simulink model "QuadCopter"  (R2016a)
settings: Solver=ode23t  StartTime=0.0  StopTime=12  FixedStep=0.001  RelTol=1e-5
InitFcn:
  | %load QuadCopterParameters
values from neighbouring files (symbols this model uses):
  Mass = 0.458    [QuadCopterParameters_m.m]
  motorCoeffs = [0.00010909388854752541 0.0075590948720063037 0.09060950915942291                 ]    [QuadCopterParameters_m.m]
undefined symbols (not defined in the file or in its folder): dc, g, Motor_F, Mxfactor, Myfactor, Qlx, Qly
libraries: Lib_Sensors x3, aerolibobsolete x1, simulink x1
settings Model: Creator=rruff  LastModifiedBy=Administrator
settings DataIOCC: LimitDataPoints=on  SaveFormat=Array  SaveOutput=off  SaveTime=off
settings OptimizationCC: DefaultParameterBehavior=Inlined  ExpressionDepthLimit=2147483647
settings DebuggingCC: SignalInfNanChecking=error  AlgebraicLoopMsg=error  UnderspecifiedInitializationDetection=Classic  MergeDetectMultiDrivingBlocksExec=none  MultiTaskDSMMsg=warning  MultiTaskCondExecSysMsg=none  FcnCallInpInsideContextMsg=EnableAllAsWarning  UnconnectedInputMsg=none  UnconnectedOutputMsg=none  UnconnectedLineMsg=none  StateNameClashWarn=warning
settings HardwareCC: ProdBitPerPointer=32  ProdLargestAtomicFloat=None  ProdIntDivRoundTo=Undefined  ProdEndianess=Unspecified  ProdWordSize=32  ProdHWDeviceType=Generic->32-bit Embedded Processor
settings ModelReferenceCC: ModelReferenceNumInstancesAllowed=Single  PropagateSignalLabelsOutOfModel=off
settings ConfigComp: CovModelRefEnable=Off  CovSFcnEnable=off
settings SimscapeCC: SelectedTab=SimMechanics2G
settings SimMechanicsCC: VisOnUpdateDiagram=on  VisDuringSimulation=on  FramesToBeSkipped=10  AnimationDelay=0  LastVizWinPosition=[1022 659 560 420]  CamPosition=[10.2752;-3.21889;-2.95529;]  CamTarget=[0;-2.23517e-09;-0.0242675;]  CamUpVector=[-0.23308;0.133123;-0.963303;]  CamHeight=0.224542  VisBackgroundColor=[0.9;0.9;0.95;]  DefaultBodyColor=[1;0;0;]
settings ConfigurationSet: Description=SimMechanics 2G
settings ExplorerConfigSet: SimMechanicsOpenEditorOnUpdate=off

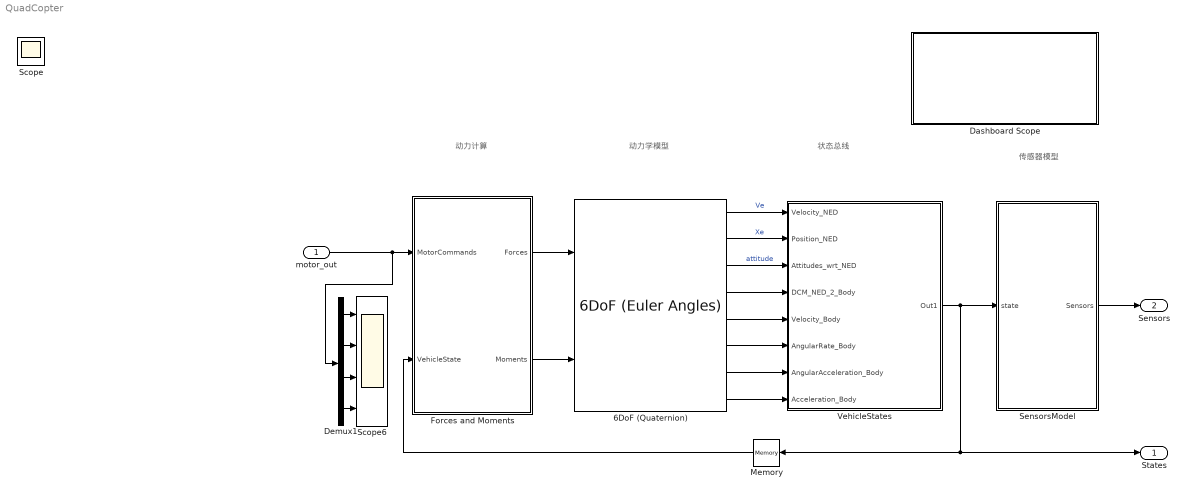
== system QuadCopter ==
  note: 传感器模型
  note: 状态总线
  note: 动力学模型
  note: 动力计算
  motor_out : Inport  PortDimensions=[4,1]
  6DoF (Quaternion) : aerolibobsolete/6DoF (Euler Angles)  units=Metric (MKS)  mtype=Fixed  rep=Quaternion  xme_0=[0 0 0]  Vm_0=[0 0 0]  eul_0=[0 0 0]  pm_0=[0 0 0]  mass_0=Mass  mass_e=0  mass_f=0  inertia=MomentInertiaTensor  inertia_e=eye(3)  inertia_f=eye(3)  k_quat=1.0
  Dashboard Scope : Subsystem  DialogController=hmiCreateDDGDialog  IsWebBlock=on  mask(MWDashboardBlock){webBlockId=dbd7d4e6-1bb4-4b4b-bc68-27a6a6e553e4, webBlockType=sdiscope, ShowInitialText=on, HMISrcModelName=QuadCopter}
      mask prompts: webBlockId "WebBlock Id"; webBlockType "WebBlock Type"; HMISrcModelName "Source Model"
      mask Help: helpview([docroot '/mapfiles/simulink.map'], 'hmi_scope')
      mask Display:
      | if strcmp(get_param(bdroot(gcb),'BlockDiagramType'), 'library')
      |     image([(matlabroot) '/toolbox/simulink/hmi/icons/DashboardScope.png']);
      | end
  Demux1 : Demux
  Forces and Moments : Subsystem  TreatAsAtomicUnit=on
  Memory : Memory
  Scope6 : Scope  NumInputPorts=4
  SensorsModel : Subsystem
  VehicleStates : Subsystem
  States : Outport  OutDataTypeStr=Bus: VehicleStates
  Sensors : Outport  Port=2  OutDataTypeStr=Bus: Sensors
  Scope : Scope
  wires:
  6DoF (Quaternion)/6 -> VehicleStates/6(AngularRate_Body)
  6DoF (Quaternion)/8 -> VehicleStates/8(Acceleration_Body)
  6DoF (Quaternion)/4 -> VehicleStates/4(DCM_NED_2_Body)
  6DoF (Quaternion)/5 -> VehicleStates/5(Velocity_Body)
  6DoF (Quaternion)/7 -> VehicleStates/7(AngularAcceleration_Body)
  6DoF (Quaternion)/3 -> VehicleStates/3(Attitudes_wrt_NED)  "attitude"
  6DoF (Quaternion)/1 -> VehicleStates/1(Velocity_NED)  "Ve"
  VehicleStates/1(Out1) -> SensorsModel/1(state), States/1, Memory/1
  6DoF (Quaternion)/2 -> VehicleStates/2(Position_NED)  "Xe"
  Memory/1 -> Forces and Moments/2(VehicleState)
  Forces and Moments/1(Forces) -> 6DoF (Quaternion)/1
  Forces and Moments/2(Moments) -> 6DoF (Quaternion)/2
  Demux1/1 -> Scope6/1
  Demux1/2 -> Scope6/2
  Demux1/3 -> Scope6/3
  Demux1/4 -> Scope6/4
  motor_out/1 -> Demux1/1, Forces and Moments/1(MotorCommands)
  SensorsModel/1(Sensors) -> Sensors/1

== system QuadCopter/Dashboard Scope ==

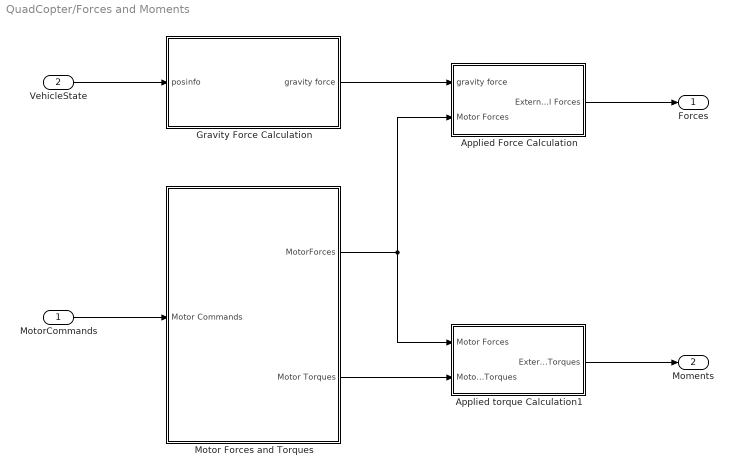
== system QuadCopter/Forces and Moments ==
  MotorCommands : Inport
  VehicleState : Inport  Port=2
  Applied Force Calculation : Subsystem
  Applied torque Calculation1 : Subsystem
  Gravity Force Calculation : Subsystem
  Motor Forces and Torques : Subsystem
  Forces : Outport
  Moments : Outport  Port=2
  wires:
  Motor Forces and Torques/1(MotorForces) -> Applied torque Calculation1/1(Motor Forces), Applied Force Calculation/2(Motor Forces)
  Applied Force Calculation/1(External Forces) -> Forces/1
  Motor Forces and Torques/2(Motor Torques) -> Applied torque Calculation1/2(Motor Torques)
  Applied torque Calculation1/1(External Torques) -> Moments/1
  MotorCommands/1 -> Motor Forces and Torques/1(Motor Commands)
  VehicleState/1 -> Gravity Force Calculation/1(posinfo)
  Gravity Force Calculation/1(gravity force) -> Applied Force Calculation/1(gravity force)

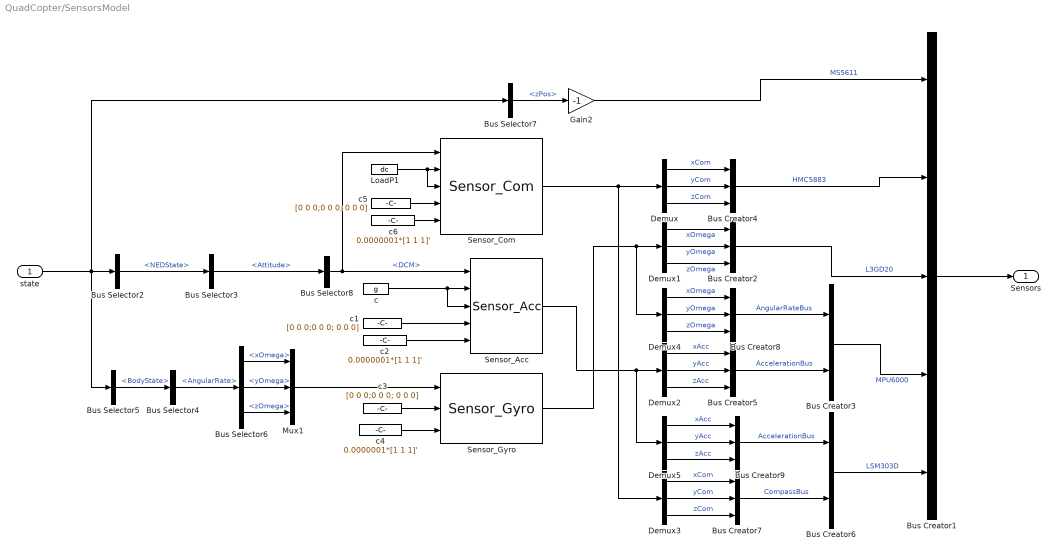
== system QuadCopter/SensorsModel ==
  state : Inport
  Bus Creator1 : BusCreator  Inputs=5  OutDataTypeStr=Bus: Sensors  NonVirtualBus=on
  Bus Creator2 : BusCreator  Inputs=3  OutDataTypeStr=Bus: AngularRateBus  NonVirtualBus=on
  Bus Creator3 : BusCreator  Inputs=2  OutDataTypeStr=Bus: MPU6000  NonVirtualBus=on
  Bus Creator4 : BusCreator  Inputs=3  OutDataTypeStr=Bus: CompassBus  NonVirtualBus=on
  Bus Creator5 : BusCreator  Inputs=3  OutDataTypeStr=Bus: AccelerationBus  NonVirtualBus=on
  Bus Creator6 : BusCreator  Inputs=2  OutDataTypeStr=Bus: LSM303D  NonVirtualBus=on
  Bus Creator7 : BusCreator  Inputs=3  OutDataTypeStr=Bus: CompassBus  NonVirtualBus=on
  Bus Creator8 : BusCreator  Inputs=3  OutDataTypeStr=Bus: AngularRateBus  NonVirtualBus=on
  Bus Creator9 : BusCreator  Inputs=3  OutDataTypeStr=Bus: AccelerationBus  NonVirtualBus=on
  Bus Selector2 : BusSelector  OutputSignals=NEDState
  Bus Selector3 : BusSelector  OutputSignals=Attitude
  Bus Selector4 : BusSelector  OutputSignals=AngularRate
  Bus Selector5 : BusSelector  OutputSignals=BodyState
  Bus Selector6 : BusSelector  OutputSignals=xOmega,yOmega,zOmega
  Bus Selector7 : BusSelector  OutputSignals=NEDState.Position.zPos
  Bus Selector8 : BusSelector  OutputSignals=DCM
  Demux{,1..5} (6 alike) : Demux  Outputs=3
  Gain2 : Gain  Gain=-1
  LoadP1 : Constant  Value=dc  SampleTime=0
  Mux1 : Mux  Inputs=3
  Sensor_Acc : Lib_Sensors/Sensor_Acc
  Sensor_Com : Lib_Sensors/Sensor_Com
  Sensor_Gyro : Lib_Sensors/Sensor_Gyro
  c : Constant  Value=g  SampleTime=0
  c1 : Constant  Value=[0 0 0;0 0 0; 0 0 0]  SampleTime=0
  c2 : Constant  Value=0.0000001*[1 1 1]'  SampleTime=0
  c3 : Constant  Value=[0 0 0;0 0 0; 0 0 0]  SampleTime=0
  c4 : Constant  Value=0.0000001*[1 1 1]'  SampleTime=0
  c5 : Constant  Value=[0 0 0;0 0 0; 0 0 0]  SampleTime=0
  c6 : Constant  Value=0.0000001*[1 1 1]'  SampleTime=0
  Sensors : Outport  OutDataTypeStr=Bus: Sensors
  wires:
  state/1 -> Bus Selector2/1, Bus Selector7/1, Bus Selector5/1
  Bus Selector2/1 -> Bus Selector3/1  "<NEDState>"
  Bus Selector5/1 -> Bus Selector4/1  "<BodyState>"
  Bus Selector4/1 -> Bus Selector6/1  "<AngularRate>"
  LoadP1/1 -> Sensor_Com/3, Sensor_Com/2
  Bus Selector6/2 -> Mux1/2  "<yOmega>"
  Bus Selector6/3 -> Mux1/3  "<zOmega>"
  Bus Selector3/1 -> Bus Selector8/1  "<Attitude>"
  Bus Selector6/1 -> Mux1/1  "<xOmega>"
  Gain2/1 -> Bus Creator1/1  "MS5611"
  Bus Creator3/1 -> Bus Creator1/4  "MPU6000"
  Bus Creator6/1 -> Bus Creator1/5  "LSM303D"
  Demux/1 -> Bus Creator4/1  "xCom"
  Demux/2 -> Bus Creator4/2  "yCom"
  Demux/3 -> Bus Creator4/3  "zCom"
  Sensor_Com/1 -> Demux3/1, Demux/1
  Demux1/1 -> Bus Creator2/1  "xOmega"
  Demux1/2 -> Bus Creator2/2  "yOmega"
  Demux1/3 -> Bus Creator2/3  "zOmega"
  Sensor_Gyro/1 -> Demux1/1, Demux4/1
  Bus Creator5/1 -> Bus Creator3/2  "AccelerationBus"
  Demux2/1 -> Bus Creator5/1  "xAcc"
  Demux2/2 -> Bus Creator5/2  "yAcc"
  Demux2/3 -> Bus Creator5/3  "zAcc"
  Bus Creator2/1 -> Bus Creator1/3  "L3GD20"
  Bus Creator4/1 -> Bus Creator1/2  "HMC5883"
  Demux3/1 -> Bus Creator7/1  "xCom"
  Demux3/2 -> Bus Creator7/2  "yCom"
  Demux3/3 -> Bus Creator7/3  "zCom"
  Bus Creator7/1 -> Bus Creator6/2  "CompassBus"
  Bus Creator1/1 -> Sensors/1
  Demux4/1 -> Bus Creator8/1  "xOmega"
  Demux4/2 -> Bus Creator8/2  "yOmega"
  Demux4/3 -> Bus Creator8/3  "zOmega"
  Bus Creator8/1 -> Bus Creator3/1  "AngularRateBus"
  Demux5/1 -> Bus Creator9/1  "xAcc"
  Demux5/2 -> Bus Creator9/2  "yAcc"
  Demux5/3 -> Bus Creator9/3  "zAcc"
  Bus Creator9/1 -> Bus Creator6/1  "AccelerationBus"
  Bus Selector7/1 -> Gain2/1  "<zPos>"
  c1/1 -> Sensor_Acc/4
  c/1 -> Sensor_Acc/3, Sensor_Acc/2
  c2/1 -> Sensor_Acc/5
  Bus Selector8/1 -> Sensor_Com/1, Sensor_Acc/1  "<DCM>"
  Sensor_Acc/1 -> Demux5/1, Demux2/1
  c3/1 -> Sensor_Gyro/2
  c4/1 -> Sensor_Gyro/3
  Mux1/1 -> Sensor_Gyro/1
  c5/1 -> Sensor_Com/4
  c6/1 -> Sensor_Com/5

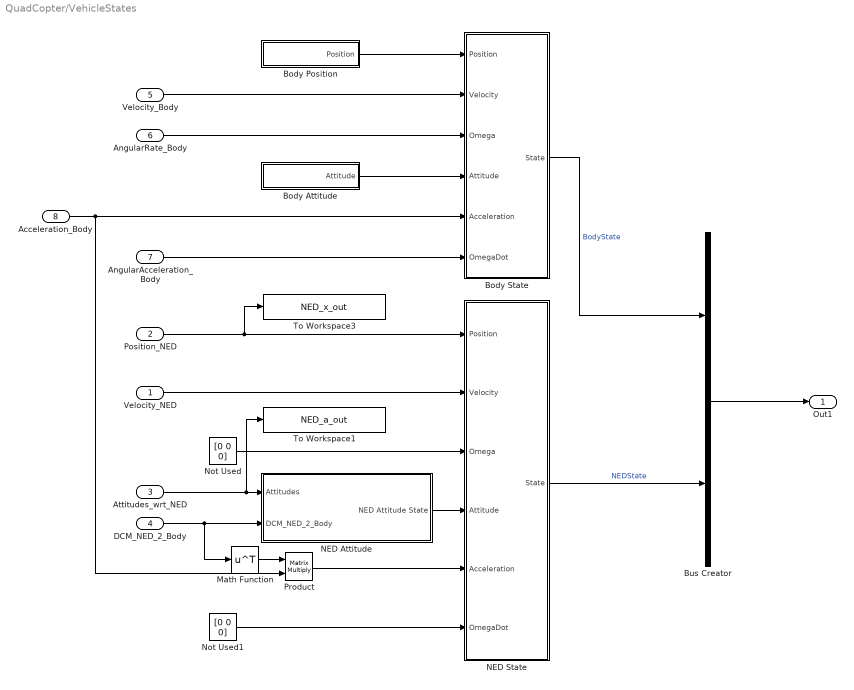
== system QuadCopter/VehicleStates ==
  Velocity_NED : Inport
  Position_NED : Inport  Port=2
  Attitudes_wrt_NED : Inport  Port=3
  DCM_NED_2_Body : Inport  Port=4
  Velocity_Body : Inport  Port=5
  AngularRate_Body : Inport  Port=6
  AngularAcceleration_Body : Inport  Port=7
  Acceleration_Body : Inport  Port=8
  Body Attitude : Subsystem
  Body Position : Subsystem
  Body State : Subsystem
  Bus Creator : BusCreator  Inputs=2  OutDataTypeStr=Bus: VehicleStates  NonVirtualBus=on
  Math Function : Math  Operator=transpose  SaturateOnIntegerOverflow=on
  NED Attitude : Subsystem
  NED State : Subsystem
  Not Used : Constant  Value=[0 0 0]
  Not Used1 : Constant  Value=[0 0 0]
  Product : Product  Multiplication=Matrix(*)
  To Workspace1 : ToWorkspace  VariableName=NED_a_out  SaveFormat=Structure  SampleTime=-1
  To Workspace3 : ToWorkspace  VariableName=NED_x_out  SaveFormat=Structure  SampleTime=-1
  Out1 : Outport
  wires:
  Bus Creator/1 -> Out1/1
  Velocity_NED/1 -> NED State/2(Velocity)
  NED Attitude/1(NED Attitude State) -> NED State/4(Attitude)
  Position_NED/1 -> To Workspace3/1, NED State/1(Position)
  Attitudes_wrt_NED/1 -> To Workspace1/1, NED Attitude/1(Attitudes)
  NED State/1(State) -> Bus Creator/2  "NEDState"
  Body State/1(State) -> Bus Creator/1  "BodyState"
  Body Attitude/1(Attitude) -> Body State/4(Attitude)
  DCM_NED_2_Body/1 -> Math Function/1, NED Attitude/2(DCM_NED_2_Body)
  Acceleration_Body/1 -> Product/2, Body State/5(Acceleration)
  AngularAcceleration_Body/1 -> Body State/6(OmegaDot)
  Velocity_Body/1 -> Body State/2(Velocity)
  Body Position/1(Position) -> Body State/1(Position)
  AngularRate_Body/1 -> Body State/3(Omega)
  Not Used/1 -> NED State/3(Omega)
  Not Used1/1 -> NED State/6(OmegaDot)
  Product/1 -> NED State/5(Acceleration)
  Math Function/1 -> Product/1

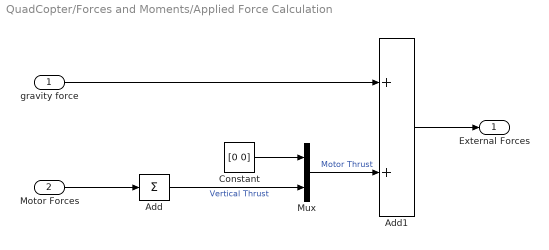
== system QuadCopter/Forces and Moments/Applied Force Calculation ==
  gravity force : Inport
  Motor Forces : Inport  Port=2
  Add : Sum  Inputs=+
  Add1 : Sum
  Constant : Constant  Value=[0 0]
  Mux : Mux  Inputs=2
  External Forces : Outport
  wires:
  Add/1 -> Mux/2  "Vertical Thrust"
  Constant/1 -> Mux/1
  Add1/1 -> External Forces/1
  Motor Forces/1 -> Add/1
  Mux/1 -> Add1/2  "Motor Thrust"
  gravity force/1 -> Add1/1

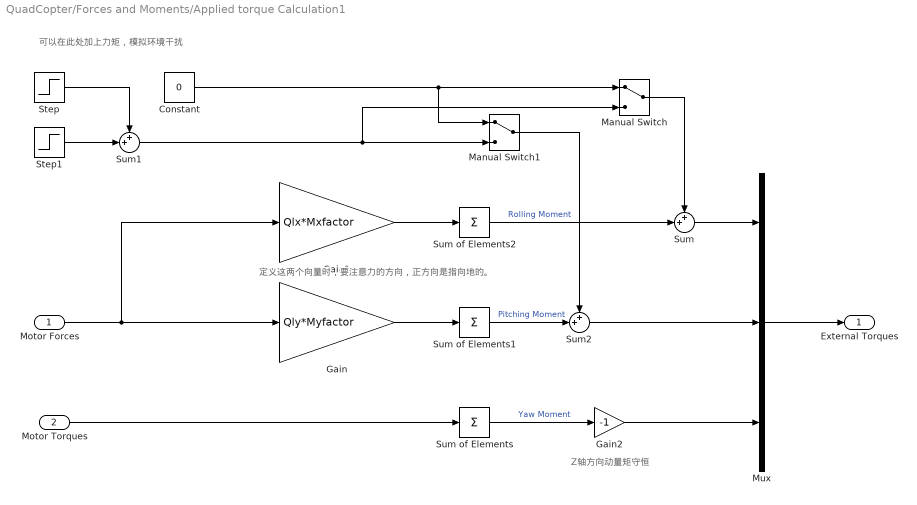
== system QuadCopter/Forces and Moments/Applied torque Calculation1 ==
  note: Z轴方向动量矩守恒
  note: 定义这两个向量时，要注意力的方向，正方向是指向地的。
  note: 可以在此处加上力矩，模拟环境干扰
  Motor Forces : Inport
  Motor Torques : Inport  Port=2
  Constant : Constant  Value=0
  Gain : Gain  Gain=Qly*Myfactor
  Gain1 : Gain  Gain=Qlx*Mxfactor
  Gain2 : Gain  Gain=-1
  Manual Switch : ManualSwitch
  Manual Switch1 : ManualSwitch
  Mux : Mux  Inputs=3
  Step : Step  Time=5  SampleTime=0
  Step1 : Step  Time=5.01  After=-1  SampleTime=0
  Sum : Sum  Inputs=++|
  Sum of Elements : Sum  Inputs=+
  Sum of Elements1 : Sum  Inputs=+
  Sum of Elements2 : Sum  Inputs=+
  Sum1 : Sum  Inputs=++|
  Sum2 : Sum  Inputs=++|
  External Torques : Outport
  wires:
  Sum of Elements/1 -> Gain2/1  "Yaw Moment"
  Motor Forces/1 -> Gain/1, Gain1/1
  Gain/1 -> Sum of Elements1/1
  Gain1/1 -> Sum of Elements2/1
  Mux/1 -> External Torques/1
  Sum/1 -> Mux/1
  Sum of Elements2/1 -> Sum/2  "Rolling Moment"
  Step1/1 -> Sum1/2
  Step/1 -> Sum1/1
  Sum2/1 -> Mux/2
  Sum of Elements1/1 -> Sum2/2  "Pitching Moment"
  Constant/1 -> Manual Switch1/1, Manual Switch/1
  Manual Switch/1 -> Sum/1
  Manual Switch1/1 -> Sum2/1
  Sum1/1 -> Manual Switch/2, Manual Switch1/2
  Motor Torques/1 -> Sum of Elements/1
  Gain2/1 -> Mux/3

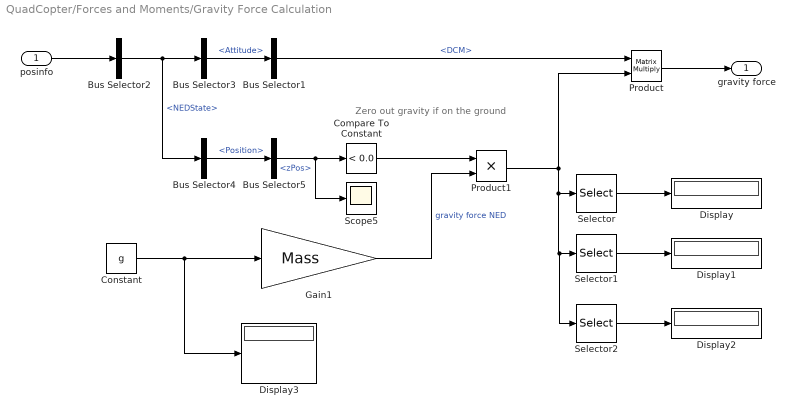
== system QuadCopter/Forces and Moments/Gravity Force Calculation ==
  note: Zero out gravity if on the ground
  posinfo : Inport
  Bus Selector1 : BusSelector  OutputSignals=DCM
  Bus Selector2 : BusSelector  OutputSignals=NEDState
  Bus Selector3 : BusSelector  OutputSignals=Attitude
  Bus Selector4 : BusSelector  OutputSignals=Position
  Bus Selector5 : BusSelector  OutputSignals=zPos
  Compare To Constant : simulink/Logic and Bit Operations/Compare To Constant  relop=<  const=0.0  OutDataTypeStr=boolean
  Constant : Constant  Value=g
  Display{,1..3} (4 alike) : Display
  Gain1 : Gain  Gain=Mass
  Product : Product  Multiplication=Matrix(*)
  Product1 : Product
  Scope5 : Scope
  Selector : Selector  InputPortWidth=3  IndexOptions=Index vector (dialog)  Indices=[1]  OutputSizes=1
  Selector1 : Selector  InputPortWidth=3  IndexOptions=Index vector (dialog)  Indices=[2]  OutputSizes=1
  Selector2 : Selector  InputPortWidth=3  IndexOptions=Index vector (dialog)  Indices=[3]  OutputSizes=1
  gravity force : Outport
  wires:
  Bus Selector3/1 -> Bus Selector1/1  "<Attitude>"
  Bus Selector2/1 -> Bus Selector4/1, Bus Selector3/1  "<NEDState>"
  posinfo/1 -> Bus Selector2/1
  Bus Selector1/1 -> Product/1  "<DCM>"
  Constant/1 -> Display3/1, Gain1/1
  Gain1/1 -> Product1/2  "gravity force NED"
  Product/1 -> gravity force/1
  Bus Selector4/1 -> Bus Selector5/1  "<Position>"
  Bus Selector5/1 -> Scope5/1, Compare To Constant/1  "<zPos>"
  Product1/1 -> Product/2, Selector2/1, Selector1/1, Selector/1
  Compare To Constant/1 -> Product1/1
  Selector/1 -> Display/1
  Selector1/1 -> Display1/1
  Selector2/1 -> Display2/1

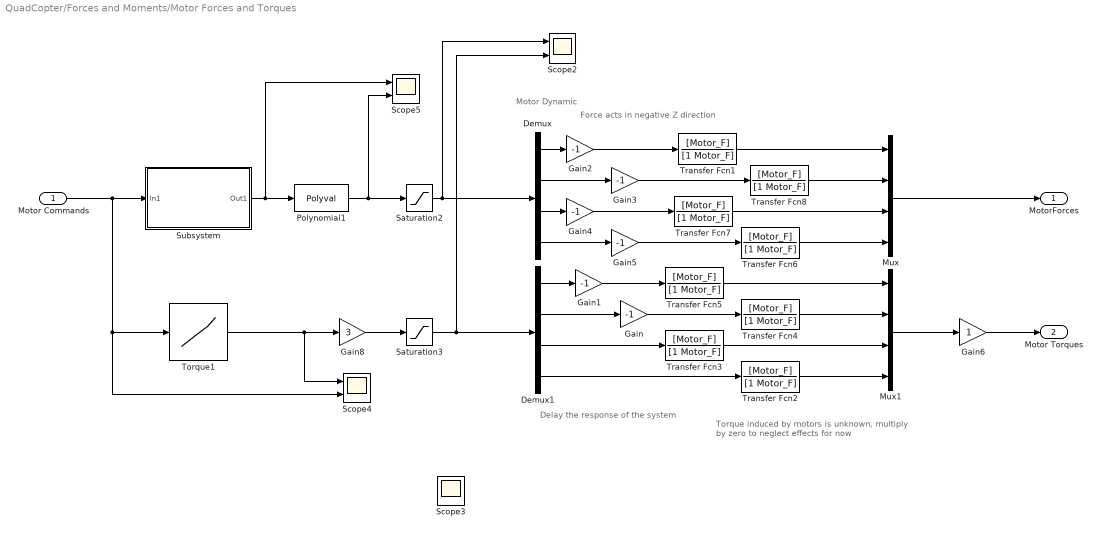
== system QuadCopter/Forces and Moments/Motor Forces and Torques ==
  note: Motor Dynamic
  note: Force acts in negative Z direction
  note: Delay the response of the system
  note: Torque induced by motors is unknown,
      | multiply by zero to neglect effects for now
  Motor Commands : Inport
  Demux : Demux
  Demux1 : Demux
  Gain{,1..5} (6 alike) : Gain  Gain=-1
  Gain6 : Gain
  Gain8 : Gain  Gain=3
  Mux : Mux
  Mux1 : Mux
  Polynomial1 : Polyval  Coefs=motorCoeffs
  Saturation2 : Saturate  UpperLimit=8.1*4  LowerLimit=0
  Saturation3 : Saturate  UpperLimit=0.189*3  LowerLimit=0
  Scope{2..5} (4 alike) : Scope  NumInputPorts=2
  Subsystem : Subsystem
  Torque1 : Lookup_n-D  NumberOfTableDimensions=1  BreakpointsForDimension1="[1160  1300  1389  1500   1600  1720  1824]"  Table="0.00980665*0.3048*[0        10    20    35     42    58    63]"  ExtrapMethod=Clip  UseLastTableValue=on  RndMeth=Simplest  InputSameDT=on
  Transfer Fcn{1..8} (8 alike) : TransferFcn  Numerator=[Motor_F]  Denominator=[1 Motor_F]
  MotorForces : Outport
  Motor Torques : Outport  Port=2
  wires:
  Transfer Fcn2/1 -> Mux1/4
  Transfer Fcn7/1 -> Mux/3
  Transfer Fcn5/1 -> Mux1/1
  Transfer Fcn4/1 -> Mux1/2
  Transfer Fcn1/1 -> Mux/1
  Gain5/1 -> Transfer Fcn6/1
  Transfer Fcn6/1 -> Mux/4
  Transfer Fcn3/1 -> Mux1/3
  Transfer Fcn8/1 -> Mux/2
  Saturation2/1 -> Scope2/1, Demux/1
  Gain4/1 -> Transfer Fcn7/1
  Gain3/1 -> Transfer Fcn8/1
  Gain2/1 -> Transfer Fcn1/1
  Demux/4 -> Gain5/1
  Demux/3 -> Gain4/1
  Demux/2 -> Gain3/1
  Demux/1 -> Gain2/1
  Mux/1 -> MotorForces/1
  Mux1/1 -> Gain6/1
  Gain6/1 -> Motor Torques/1
  Demux1/1 -> Gain1/1
  Demux1/2 -> Gain/1
  Demux1/3 -> Transfer Fcn3/1
  Demux1/4 -> Transfer Fcn2/1
  Torque1/1 -> Scope4/1, Gain8/1
  Polynomial1/1 -> Scope5/2, Saturation2/1
  Saturation3/1 -> Scope2/2, Demux1/1
  Gain8/1 -> Saturation3/1
  Subsystem/1(Out1) -> Scope5/1, Polynomial1/1
  Motor Commands/1 -> Scope4/2, Torque1/1, Subsystem/1(In1)
  Gain1/1 -> Transfer Fcn5/1
  Gain/1 -> Transfer Fcn4/1

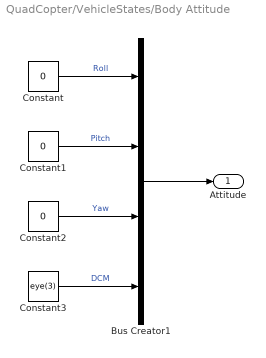
== system QuadCopter/VehicleStates/Body Attitude ==
  Bus Creator1 : BusCreator  Inputs=4  OutDataTypeStr=Bus: AttitudeBus  NonVirtualBus=on
  Constant : Constant  Value=0
  Constant1 : Constant  Value=0
  Constant2 : Constant  Value=0
  Constant3 : Constant  Value=eye(3)
  Attitude : Outport
  wires:
  Constant/1 -> Bus Creator1/1  "Roll"
  Bus Creator1/1 -> Attitude/1
  Constant1/1 -> Bus Creator1/2  "Pitch"
  Constant2/1 -> Bus Creator1/3  "Yaw"
  Constant3/1 -> Bus Creator1/4  "DCM"

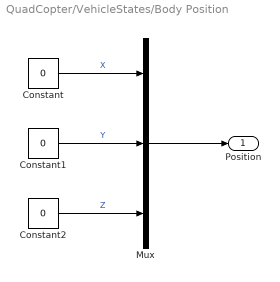
== system QuadCopter/VehicleStates/Body Position ==
  Constant : Constant  Value=0
  Constant1 : Constant  Value=0
  Constant2 : Constant  Value=0
  Mux : Mux  Inputs=3
  Position : Outport
  wires:
  Constant2/1 -> Mux/3  "Z"
  Constant1/1 -> Mux/2  "Y"
  Constant/1 -> Mux/1  "X"
  Mux/1 -> Position/1

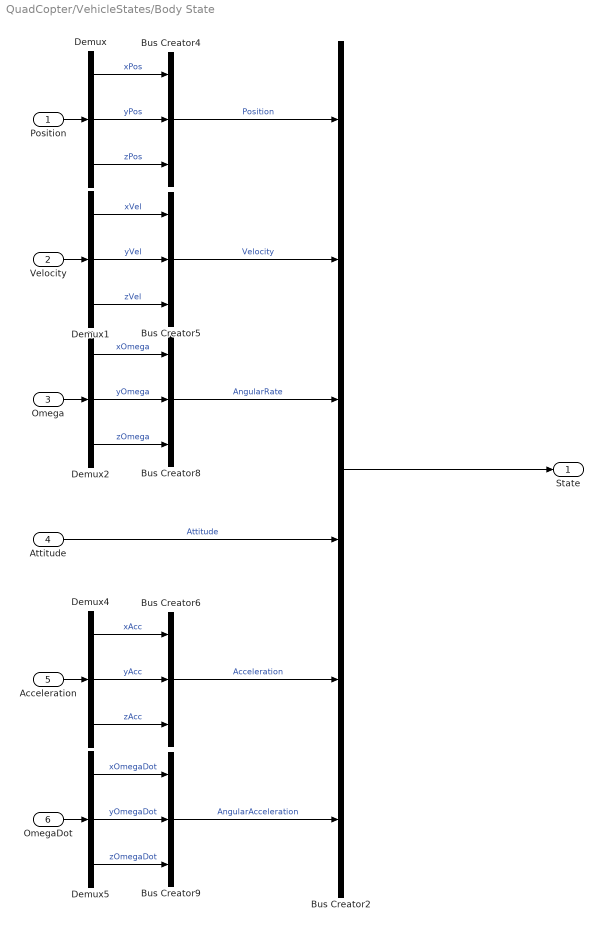
== system QuadCopter/VehicleStates/Body State ==
  Position : Inport
  Velocity : Inport  Port=2
  Omega : Inport  Port=3
  Attitude : Inport  Port=4
  Acceleration : Inport  Port=5
  OmegaDot : Inport  Port=6
  Bus Creator2 : BusCreator  Inputs=6  OutDataTypeStr=Bus: States  NonVirtualBus=on
  Bus Creator4 : BusCreator  Inputs=3  OutDataTypeStr=Bus: PositionBus  NonVirtualBus=on
  Bus Creator5 : BusCreator  Inputs=3  OutDataTypeStr=Bus: VelocityBus  NonVirtualBus=on
  Bus Creator6 : BusCreator  Inputs=3  OutDataTypeStr=Bus: AccelerationBus  NonVirtualBus=on
  Bus Creator8 : BusCreator  Inputs=3  OutDataTypeStr=Bus: AngularRateBus  NonVirtualBus=on
  Bus Creator9 : BusCreator  Inputs=3  OutDataTypeStr=Bus: AngularAccelerationBus  NonVirtualBus=on
  Demux{,1..2,4..5} (5 alike) : Demux  Outputs=3
  State : Outport  OutDataTypeStr=Bus: States
  wires:
  Demux/1 -> Bus Creator4/1  "xPos"
  Demux/2 -> Bus Creator4/2  "yPos"
  Demux/3 -> Bus Creator4/3  "zPos"
  Demux1/1 -> Bus Creator5/1  "xVel"
  Demux1/2 -> Bus Creator5/2  "yVel"
  Demux1/3 -> Bus Creator5/3  "zVel"
  Demux2/1 -> Bus Creator8/1  "xOmega"
  Demux2/2 -> Bus Creator8/2  "yOmega"
  Demux2/3 -> Bus Creator8/3  "zOmega"
  Demux4/1 -> Bus Creator6/1  "xAcc"
  Demux4/2 -> Bus Creator6/2  "yAcc"
  Demux4/3 -> Bus Creator6/3  "zAcc"
  Demux5/1 -> Bus Creator9/1  "xOmegaDot"
  Demux5/2 -> Bus Creator9/2  "yOmegaDot"
  Demux5/3 -> Bus Creator9/3  "zOmegaDot"
  Bus Creator4/1 -> Bus Creator2/1  "Position"
  Bus Creator5/1 -> Bus Creator2/2  "Velocity"
  Bus Creator8/1 -> Bus Creator2/3  "AngularRate"
  Attitude/1 -> Bus Creator2/4  "Attitude"
  Bus Creator6/1 -> Bus Creator2/5  "Acceleration"
  Bus Creator9/1 -> Bus Creator2/6  "AngularAcceleration"
  Position/1 -> Demux/1
  Velocity/1 -> Demux1/1
  Omega/1 -> Demux2/1
  Bus Creator2/1 -> State/1
  Acceleration/1 -> Demux4/1
  OmegaDot/1 -> Demux5/1

== system QuadCopter/VehicleStates/NED Attitude ==
  Attitudes : Inport
  DCM_NED_2_Body : Inport  Port=2
  Bus Creator7 : BusCreator  Inputs=4  OutDataTypeStr=Bus: AttitudeBus  NonVirtualBus=on
  Demux3 : Demux  Outputs=3
  NED Attitude State : Outport
  wires:
  Attitudes/1 -> Demux3/1
  DCM_NED_2_Body/1 -> Bus Creator7/4  "DCM"
  Demux3/1 -> Bus Creator7/1  "Roll"
  Bus Creator7/1 -> NED Attitude State/1  "Attitude"
  Demux3/3 -> Bus Creator7/3  "Yaw"
  Demux3/2 -> Bus Creator7/2  "Pitch"

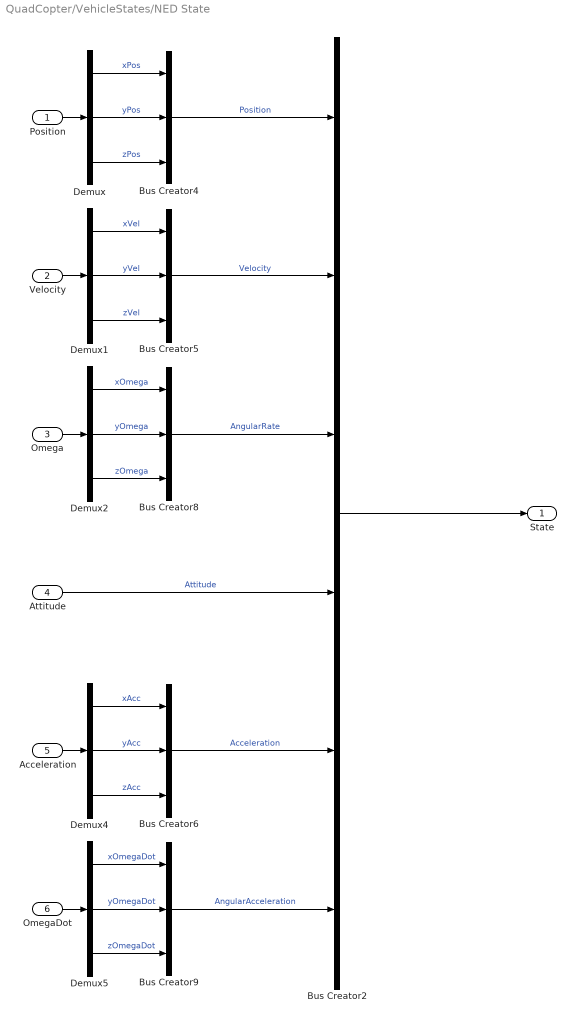
== system QuadCopter/VehicleStates/NED State ==
  Position : Inport
  Velocity : Inport  Port=2
  Omega : Inport  Port=3
  Attitude : Inport  Port=4
  Acceleration : Inport  Port=5
  OmegaDot : Inport  Port=6
  Bus Creator2 : BusCreator  Inputs=6  OutDataTypeStr=Bus: States  NonVirtualBus=on
  Bus Creator4 : BusCreator  Inputs=3  OutDataTypeStr=Bus: PositionBus  NonVirtualBus=on
  Bus Creator5 : BusCreator  Inputs=3  OutDataTypeStr=Bus: VelocityBus  NonVirtualBus=on
  Bus Creator6 : BusCreator  Inputs=3  OutDataTypeStr=Bus: AccelerationBus  NonVirtualBus=on
  Bus Creator8 : BusCreator  Inputs=3  OutDataTypeStr=Bus: AngularRateBus  NonVirtualBus=on
  Bus Creator9 : BusCreator  Inputs=3  OutDataTypeStr=Bus: AngularAccelerationBus  NonVirtualBus=on
  Demux{,1..2,4..5} (5 alike) : Demux  Outputs=3
  State : Outport  OutDataTypeStr=Bus: States
  wires:
  Demux/1 -> Bus Creator4/1  "xPos"
  Demux/2 -> Bus Creator4/2  "yPos"
  Demux/3 -> Bus Creator4/3  "zPos"
  Demux1/1 -> Bus Creator5/1  "xVel"
  Demux1/2 -> Bus Creator5/2  "yVel"
  Demux1/3 -> Bus Creator5/3  "zVel"
  Demux2/1 -> Bus Creator8/1  "xOmega"
  Demux2/2 -> Bus Creator8/2  "yOmega"
  Demux2/3 -> Bus Creator8/3  "zOmega"
  Demux4/1 -> Bus Creator6/1  "xAcc"
  Demux4/2 -> Bus Creator6/2  "yAcc"
  Demux4/3 -> Bus Creator6/3  "zAcc"
  Demux5/1 -> Bus Creator9/1  "xOmegaDot"
  Demux5/2 -> Bus Creator9/2  "yOmegaDot"
  Demux5/3 -> Bus Creator9/3  "zOmegaDot"
  Bus Creator4/1 -> Bus Creator2/1  "Position"
  Bus Creator5/1 -> Bus Creator2/2  "Velocity"
  Bus Creator8/1 -> Bus Creator2/3  "AngularRate"
  Bus Creator6/1 -> Bus Creator2/5  "Acceleration"
  Bus Creator9/1 -> Bus Creator2/6  "AngularAcceleration"
  Position/1 -> Demux/1
  Velocity/1 -> Demux1/1
  Omega/1 -> Demux2/1
  Bus Creator2/1 -> State/1
  Attitude/1 -> Bus Creator2/4  "Attitude"
  Acceleration/1 -> Demux4/1
  OmegaDot/1 -> Demux5/1

== system QuadCopter/Forces and Moments/Motor Forces and Torques/Subsystem ==
  In1 : Inport
  Gain9 : Gain  Gain=1/10.0
  Sum : Sum  Inputs=-+
  throttleOffset : Constant  Value=1000
  Out1 : Outport
  wires:
  Gain9/1 -> Out1/1
  In1/1 -> Sum/2
  throttleOffset/1 -> Sum/1
  Sum/1 -> Gain9/1
